simulink model "SimuSandbox"  (R2021b)
settings: Solver=VariableStepAuto  StartTime=0.0  StopTime=10.0  RelTol=1e-3
values from neighbouring files (symbols this model uses):
  h = 0.05    [Identified_system1_data.mat]    (also in Identified_system2_data.mat; Identified_system3_data.mat; Identified_system4_data.mat; MotorID_data.mat)
  params = cell2struct([struct2cell(motorparams);struct2cell(pendparams)],[fieldnames(motorparams);fieldnames(pendparams)],1)    [A1masterMain_Measurements.m]
  sys = ss(sys.A, sys.B, eye(nx), zeros(nx,1), h)    [A1masterMain.m]    (also in A1masterMain_Measurements.m; SysIDgrey_fullParamed.m = ss(Ac,Bc,Cc,Dc); SysIDgrey_motor.m = ss(Ac,Bc,Cc,Dc); SysIDgrey_semiParamed.m = ss(Ac,Bc,Cc,Dc))
settings Model: Creator=sachi  LastModifiedBy=sachi

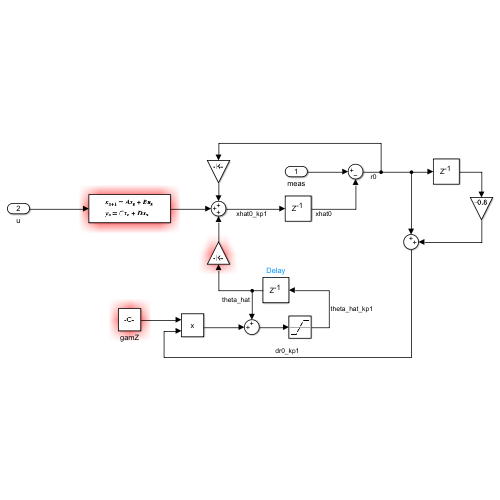
[thumbnail: Simulink's stored preview of the top-level diagram]
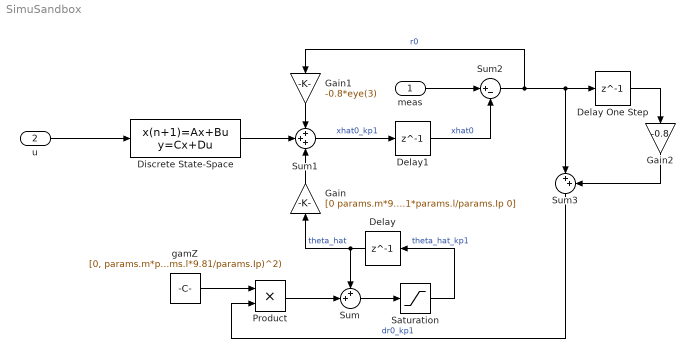
== system SimuSandbox ==
  meas : Inport
  u : Inport  Port=2
  Delay : Delay  DelayLength=1  InitialCondition=0
  Delay One Step : Delay  DelayLength=1
  Delay1 : Delay  DelayLength=1  InitialCondition=0
  Discrete State-Space : DiscreteStateSpace  A=sys.A  B=sys.B  C=sys.C  D=sys.D  SampleTime=h
  Gain : Gain  Gain=[0 params.m*9.81*params.l/params.Ip 0]
  Gain1 : Gain  Gain=-0.8*eye(3)
  Gain2 : Gain  Gain=-0.8
  Product : Product
  Saturation : Saturate  UpperLimit=deg2rad(2)  LowerLimit=-deg2rad(2)
  Sum : Sum  Inputs=++|
  Sum1 : Sum  Inputs=+++
  Sum2 : Sum  Inputs=|+-
  Sum3 : Sum  Inputs=|++
  gamZ : Constant  Value=[0, params.m*params.l*9.81/params.Ip, 0] .* 1/(1e-6 + abs(params.m*params.l*9.81/params.Ip)^2)
  wires:
  gamZ/1 -> Product/1
  Product/1 -> Sum/2
  Sum/1 -> Saturation/1
  Saturation/1 -> Delay/1  "theta_hat_kp1"
  Delay/1 -> Sum/1, Gain/1  "theta_hat"
  u/1 -> Discrete State-Space/1
  Discrete State-Space/1 -> Sum1/2
  Gain/1 -> Sum1/3
  Sum1/1 -> Delay1/1  "xhat0_kp1"
  Delay1/1 -> Sum2/2  "xhat0"
  meas/1 -> Sum2/1
  Sum2/1 -> Gain1/1, Sum3/1, Delay One Step/1  "r0"
  Gain1/1 -> Sum1/1
  Delay One Step/1 -> Gain2/1
  Gain2/1 -> Sum3/2
  Sum3/1 -> Product/2  "dr0_kp1"
